simulink model "Control_Model_2020a"  (R2020a)
settings: Solver=ode3  StartTime=0.0  StopTime=20  FixedStep=0.001  RelTol=1e-3
InitFcn:
  | init_parameters
undefined symbols (not defined in the file): Bf, Bm, Br, DiscIntNeverNeededParam, f, g, hg, i_sw, I_tire, Iz, k1, k2, k3, K_LQR, kd_beta, kd_omega, ki_beta, ki_omega, kp_beta, kp_omega, L, Lf, Lm, Lr, m, magnitude, mb, mw, Mz_K, Pn_motor, r, sigbuilder_block, Tn_motor, v_obj, vx0, w0
libraries: simulink x2, Solver_SF x1, simulink_extras x1
(part 1 of 2)
settings Model: Creator=Qian  LastModifiedBy=Administrator
settings OptimizationCC: LifeSpan=inf
settings DebuggingCC: ArithmeticOperatorsInVariantConditions=warning
settings SFSimCC: CustomCodeUndefinedFunction=UseInterfaceOnly
settings RTWCC: GenCodeOnly=on
settings CodeAppCC: StateflowObjectComments=on

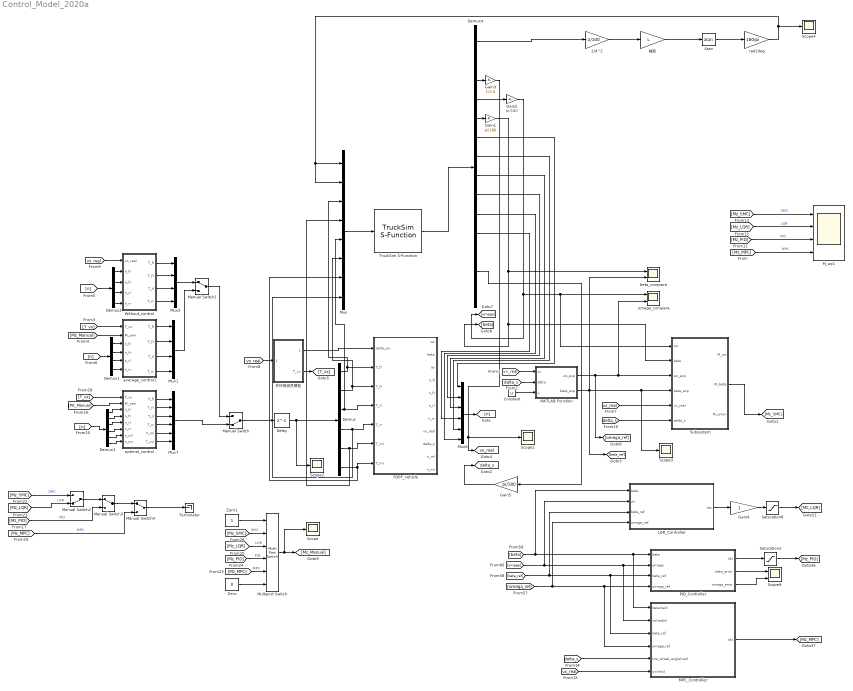
== system Control_Model_2020a ==
  2/d^2 : Gain  Gain=-2/100
  7DOF_vehicle : Subsystem
  Atan : Trigonometry  Operator=atan
  Constant : Constant  Value=u
  Delay : Delay  DelayLength=1
  Demux : Demux  Outputs=6
  Demux1 : Demux
  Demux2 : Demux
  Demux3 : Demux  Outputs=6
  Demux4 : Demux  Outputs=14
  Gain1 : Gain  Gain=pi/180
  Gain2 : Gain  Gain=pi/180
  Gain3 : Gain  Gain=1/3.6
  Gain4 : Gain
  Gain5 : Gain  Gain=pi/180
  LQR_Controller : Subsystem
  MATLAB Function : MATLAB Function  TreatAsAtomicUnit=on
  MPC_Controller : Subsystem
  M_wz1 : Scope  NumInputPorts=4
  Manual Switch : ManualSwitch  CurrentSetting=0
  Manual Switch1 : ManualSwitch
  Manual Switch2 : ManualSwitch  CurrentSetting=0
  Manual Switch3 : ManualSwitch
  Manual Switch4 : ManualSwitch
  Multiport Switch : MultiPortSwitch  Inputs=5
  Mux : Mux  Inputs=8
  Mux1 : Mux
  Mux3 : Mux
  Mux6 : Mux  Inputs=6
  Mux7 : Mux  Inputs=6
  PID_Controller : Subsystem
  Saturation2 : Saturate  UpperLimit=2000  LowerLimit=-2000
  Saturation8 : Saturate  UpperLimit=2000  LowerLimit=-2000
  Scope{,1..4} (5 alike) : Scope
  Scope9 : Scope  NumInputPorts=2
  Subsystem : Subsystem
  Terminator : Terminator
  TruckSim S-Function : Solver_SF/TruckSim S-Function  Priority=1  SIMFILE=simfile.sim
      settings: SourceProductName=TruckSim S-Function
  Without_control : Subsystem
  Zero : Constant  Value=0  OutDataTypeStr=Inherit: Inherit via back propagation
  Zero1 : Constant  OutDataTypeStr=Inherit: Inherit via back propagation
  average_control1 : Subsystem
  beta_compare : Scope  NumInputPorts=2
  omega_compare : Scope  NumInputPorts=2
  optimal_control : Subsystem
  rad2deg : Gain  Gain=180/pi
  开环驾驶员模型 : Subsystem
  轴距 : Gain  Gain=L
  tag scope: delta_s=global, vx_real=global
  wires:
  Demux2/1 -> Without_control/2(n_fl)
  Demux3/2 -> optimal_control/4(n_fr)
  [delta_s] -> MPC_Controller/5(tire_wheel_angle(rad))
  MPC_Controller/1(Mz) -> [Mz_MPC]
  Demux1/4 -> average_control1/6(n_rr)
  [n] -> Demux1/1
  [Mz_SMC] -> M_wz1/1  "SMC"
  PID_Controller/3(omega_error) -> Scope9/2
  Manual Switch/1 -> Delay/1
  MATLAB Function/2(beta_exp) -> [beta_ref], beta_compare/2, Scope3/1, Subsystem/4(beta_exp)
  average_control1/4(T_rr) -> Mux1/4
  Demux3/1 -> optimal_control/3(n_fl)
  Demux1/3 -> average_control1/5(n_rl)
  [Mz_Manual] -> average_control1/2(M_yaw)
  [n] -> Demux2/1
  average_control1/3(T_rl) -> Mux1/3
  Demux3/4 -> optimal_control/6(n_rr)
  Demux1/2 -> average_control1/4(n_fr)
  MATLAB Function/1(wz_exp) -> omega_compare/2, Subsystem/3(wz_exp), [omega_ref]
  开环驾驶员模型/1(delta_sw) -> 7DOF_vehicle/1(delta_sw)
  Demux/4 -> Mux/8, 7DOF_vehicle/5(T_rr)
  Demux/3 -> 7DOF_vehicle/4(T_rl), Mux/5
  Demux/1 -> Mux/3, 7DOF_vehicle/2(T_fl)
  Without_control/3(T_rl) -> Mux3/3
  Demux2/3 -> Without_control/4(n_rl)
  [n] -> Demux3/1
  Constant/1 -> MATLAB Function/3(u)
  optimal_control/2(T_fr) -> Mux7/2
  [vx_real] -> Without_control/1(vx_real)
  optimal_control/1(T_fl) -> Mux7/1
  Without_control/2(T_fr) -> Mux3/2
  Demux2/4 -> Without_control/5(n_rr)
  Demux2/2 -> Without_control/3(n_fr)
  Without_control/4(T_rr) -> Mux3/4
  Without_control/1(T_fl) -> Mux3/1
  Manual Switch4/1 -> Terminator/1
  average_control1/2(T_fr) -> Mux1/2
  [beta] -> LQR_Controller/1(beta), MPC_Controller/1(beta(rad)), PID_Controller/1(beta)
  Manual Switch3/1 -> Manual Switch4/1
  optimal_control/3(T_rl) -> Mux7/3
  [T_vx] -> optimal_control/1(T_vx)
  [Mz_Manual] -> optimal_control/2(M_yaw)
  [Mz_PID] -> Manual Switch3/2  "PID"
  [vx_real] -> MPC_Controller/6(vx(m/s))
  [vx_real] -> MATLAB Function/1(vx)
  [Mz_MPC] -> Manual Switch4/2  "MPC"
  [omega] -> LQR_Controller/2(wr), PID_Controller/2(omega), MPC_Controller/2(wr(rad/s))
  [vx_real] -> 开环驾驶员模型/1(vx_real)
  Saturation2/1 -> [Mz_PID]
  [Mz_SMC] -> Manual Switch2/1  "SMC"
  optimal_control/4(T_rr) -> Mux7/4
  Mux6/1 -> [n]
  Demux1/1 -> average_control1/3(n_fl)
  [T_vx] -> average_control1/1(T_vx)
  [omega_ref] -> LQR_Controller/4(omega_ref), PID_Controller/4(omega_ref), MPC_Controller/4(omega_ref)
  Mux7/1 -> Manual Switch/2
  LQR_Controller/1(Mz) -> Gain4/1
  [Mz_LQR] -> M_wz1/2  "LQR"
  PID_Controller/2(beta_error) -> Scope9/1
  [Mz_PID] -> M_wz1/3  "PID"
  Demux/2 -> Mux/6, 7DOF_vehicle/3(T_fr)
  Mux3/1 -> Manual Switch1/1
  average_control1/1(T_fl) -> Mux1/1
  [Mz_MPC] -> M_wz1/4  "MPC"
  Manual Switch2/1 -> Manual Switch3/1
  [beta_ref] -> LQR_Controller/3(beta_ref), PID_Controller/3(beta_ref), MPC_Controller/3(beta_ref)
  Mux1/1 -> Manual Switch1/2
  PID_Controller/1(Mz) -> Saturation2/1
  开环驾驶员模型/2(T_vx) -> [T_vx]
  [delta_s] -> MATLAB Function/2(delta)
  [Mz_LQR] -> Manual Switch2/2  "LQR"
  Demux3/3 -> optimal_control/5(n_rl)
  Manual Switch1/1 -> Manual Switch/1
  [Mz_SMC] -> Multiport Switch/2  "SMC"
  [Mz_MPC] -> Multiport Switch/5  "MPC"
  [Mz_PID] -> Multiport Switch/4  "PID"
  [Mz_LQR] -> Multiport Switch/3  "LQR"
  Zero/1 -> Multiport Switch/6
  Multiport Switch/1 -> Scope/1, [Mz_Manual]
  Zero1/1 -> Multiport Switch/1
  Saturation8/1 -> [Mz_LQR]
  Gain4/1 -> Saturation8/1
  Delay/1 -> Scope2/1, Demux/1
  optimal_control/5(T_ml) -> Mux7/5
  optimal_control/6(T_mr) -> Mux7/6
  Demux/5 -> Mux/4, 7DOF_vehicle/6(T_ml)
  Demux/6 -> Mux/7, 7DOF_vehicle/7(T_mr)
  Demux3/5 -> optimal_control/7(n_ml)
  Demux3/6 -> optimal_control/8(n_mr)
  TruckSim S-Function/1 -> Demux4/1
  Mux/1 -> TruckSim S-Function/1
  Demux4/4 -> Gain2/1
  Demux4/5 -> Gain1/1
  Demux4/6 -> Mux6/1
  Demux4/7 -> Mux6/5
  Demux4/8 -> Mux6/3
  Demux4/9 -> Mux6/2
  Demux4/10 -> Mux6/6
  Demux4/11 -> Mux6/4
  Demux4/3 -> Gain3/1
  2/d^2/1 -> 轴距/1
  轴距/1 -> Atan/1
  Atan/1 -> rad2deg/1
  Demux4/1 -> 2/d^2/1
  rad2deg/1 -> Scope4/1, Mux/1, Mux/2
  [delta_s] -> Subsystem/6(delta_s)
  [vx_real] -> Subsystem/5(vx_real)
  Gain3/1 -> Scope1/1, [vx_real]
  Gain1/1 -> beta_compare/1, [beta], Subsystem/2(beta)
  Gain2/1 -> [omega], Subsystem/1(wz), omega_compare/1
  Gain5/1 -> [delta_s]
  Demux4/13 -> Gain5/1
  Subsystem/2(M_beta) -> [Mz_SMC]

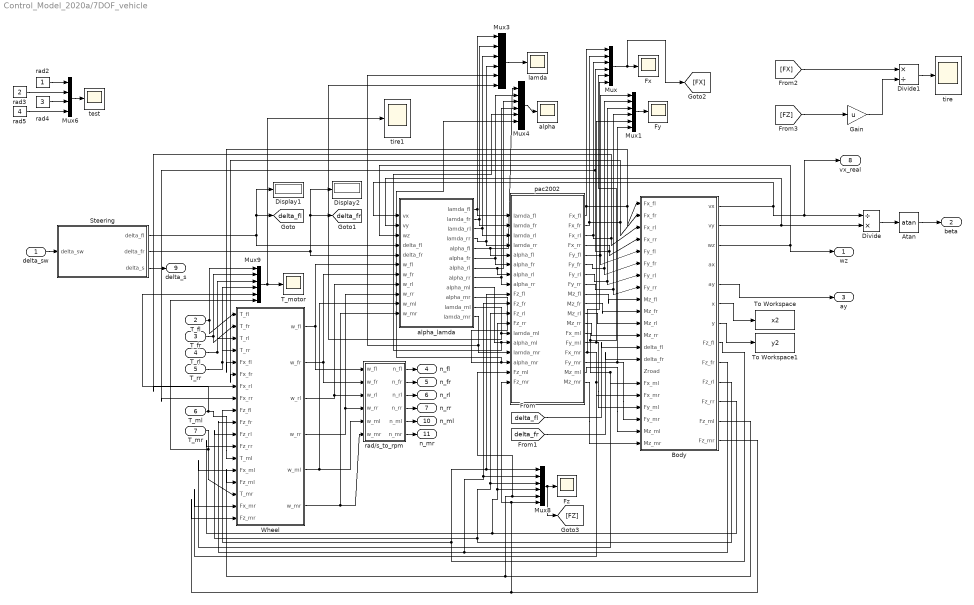
== system Control_Model_2020a/7DOF_vehicle ==
  delta_sw : Inport
  T_fl : Inport  Port=2
  T_fr : Inport  Port=3
  T_rl : Inport  Port=4
  T_rr : Inport  Port=5
  T_ml : Inport  Port=6
  T_mr : Inport  Port=7
  Atan : Trigonometry  Operator=atan
  Body : Subsystem
  Display1 : Display
  Display2 : Display
  Divide : Product  Inputs=/*
  Divide1 : Product  Inputs=*/
  Fx : Scope
  Fy : Scope
  Fz : Scope
  Gain : Gain  Gain=u
  Mux{,1,3..4,8..9} (6 alike) : Mux  Inputs=6
  Mux6 : Mux
  Steering : Subsystem
  T_motor : Scope
  To Workspace : ToWorkspace  VariableName=x2  SampleTime=-1
  To Workspace1 : ToWorkspace  VariableName=y2  SampleTime=-1
  Wheel : Subsystem
  alpha : Scope
  alpha_lamda : Subsystem
  lamda : Scope
  pac2002 : Subsystem
  rad/s_to_rpm : Subsystem
  rad2 : Constant
  rad3 : Constant  Value=2
  rad4 : Constant  Value=3
  rad5 : Constant  Value=4
  test : Scope
  tire : Scope
  tire1 : Scope
  wz : Outport
  beta : Outport  Port=2
  ay : Outport  Port=3
  n_fl : Outport  Port=4
  n_fr : Outport  Port=5
  n_rl : Outport  Port=6
  n_rr : Outport  Port=7
  vx_real : Outport  Port=8
  delta_s : Outport  Port=9
  n_ml : Outport  Port=10
  n_mr : Outport  Port=11
  tag scope: delta_fl=global, delta_fr=global
  wires:
  pac2002/12(Mz_rr) -> Body/12(Mz_rr)
  pac2002/11(Mz_rl) -> Body/11(Mz_rl)
  pac2002/10(Mz_fr) -> Body/10(Mz_fr)
  pac2002/9(Mz_fl) -> Body/9(Mz_fl)
  Atan/1 -> beta/1
  Divide/1 -> Atan/1
  T_rr/1 -> Mux9/4, Wheel/4(T_rr)
  rad/s_to_rpm/4(n_rr) -> n_rr/1
  rad/s_to_rpm/2(n_fr) -> n_fr/1
  T_rl/1 -> Mux9/3, Wheel/3(T_rl)
  Body/5(ay) -> ay/1
  Body/1(vx) -> vx_real/1, Divide/1, alpha_lamda/1(vx)
  Mux6/1 -> test/1
  Wheel/4(w_rr) -> alpha_lamda/9(w_rr), rad/s_to_rpm/4(w_rr)
  rad3/1 -> Mux6/2
  delta_sw/1 -> Steering/1(delta_sw)
  Body/2(vy) -> alpha_lamda/2(vy), Divide/2
  rad4/1 -> Mux6/3
  rad5/1 -> Mux6/4
  Mux3/1 -> lamda/1
  Mux/1 -> [FX], Fx/1
  T_fl/1 -> Mux9/1, Wheel/1(T_fl)
  Body/11(Fz_rr) -> pac2002/12(Fz_rr), Mux8/4, Wheel/12(Fz_rr)
  Mux4/1 -> alpha/1
  rad/s_to_rpm/3(n_rl) -> n_rl/1
  T_fr/1 -> Mux9/2, Wheel/2(T_fr)
  pac2002/3(Fx_rl) -> Mux/3, Body/3(Fx_rl), Wheel/7(Fx_rl)
  alpha_lamda/6(alpha_fr) -> pac2002/6(alpha_fr), Mux4/2
  Body/9(Fz_fr) -> pac2002/10(Fz_fr), Mux8/2, Wheel/10(Fz_fr)
  [delta_fr] -> Body/14(delta_fr)
  alpha_lamda/5(alpha_fl) -> pac2002/5(alpha_fl), Mux4/1
  alpha_lamda/8(alpha_rr) -> pac2002/8(alpha_rr), Mux4/4
  Wheel/1(w_fl) -> rad/s_to_rpm/1(w_fl), alpha_lamda/6(w_fl)
  Wheel/3(w_rl) -> rad/s_to_rpm/3(w_rl), alpha_lamda/8(w_rl)
  Body/10(Fz_rl) -> pac2002/11(Fz_rl), Mux8/3, Wheel/11(Fz_rl)
  Mux1/1 -> Fy/1
  rad/s_to_rpm/1(n_fl) -> n_fl/1
  alpha_lamda/7(alpha_rl) -> pac2002/7(alpha_rl), Mux4/3
  Mux8/1 -> [FZ], Fz/1
  Wheel/2(w_fr) -> rad/s_to_rpm/2(w_fr), alpha_lamda/7(w_fr)
  pac2002/8(Fy_rr) -> Body/8(Fy_rr), Mux1/4
  alpha_lamda/2(lamda_fr) -> pac2002/2(lamda_fr), Mux3/2
  pac2002/5(Fy_fl) -> Body/5(Fy_fl), Mux1/1
  pac2002/2(Fx_fr) -> Mux/2, Body/2(Fx_fr), Wheel/6(Fx_fr)
  Body/8(Fz_fl) -> pac2002/9(Fz_fl), Mux8/1, Wheel/9(Fz_fl)
  alpha_lamda/3(lamda_rl) -> pac2002/3(lamda_rl), Mux3/3
  pac2002/6(Fy_fr) -> Body/6(Fy_fr), Mux1/2
  pac2002/7(Fy_rl) -> Body/7(Fy_rl), Mux1/3
  Steering/2(delta_fr) -> alpha_lamda/5(delta_fr), Display2/1, [delta_fr]
  Steering/1(delta_fl) -> alpha_lamda/4(delta_fl), Display1/1, [delta_fl]
  alpha_lamda/4(lamda_rr) -> pac2002/4(lamda_rr), Mux3/4
  alpha_lamda/1(lamda_fl) -> Mux3/1, pac2002/1(lamda_fl)
  pac2002/1(Fx_fl) -> Mux/1, Body/1(Fx_fl), Wheel/5(Fx_fl)
  rad2/1 -> Mux6/1
  [delta_fl] -> Body/13(delta_fl)
  Body/3(wz) -> wz/1, alpha_lamda/3(wz)
  pac2002/4(Fx_rr) -> Mux/4, Wheel/8(Fx_rr), Body/4(Fx_rr)
  Body/6(x) -> To Workspace/1
  Body/7(y) -> To Workspace1/1
  [FZ] -> Gain/1
  [FX] -> Divide1/1
  Gain/1 -> Divide1/2
  Divide1/1 -> tire/1
  Mux9/1 -> tire1/1, T_motor/1
  Steering/3(delta_s) -> delta_s/1
  rad/s_to_rpm/5(n_ml) -> n_ml/1
  rad/s_to_rpm/6(n_mr) -> n_mr/1
  Wheel/5(w_ml) -> alpha_lamda/10(w_ml), rad/s_to_rpm/5(w_ml)
  Wheel/6(w_mr) -> alpha_lamda/11(w_mr), rad/s_to_rpm/6(w_mr)
  alpha_lamda/11(lamda_ml) -> Mux3/6, pac2002/13(lamda_ml)
  alpha_lamda/9(alpha_ml) -> Mux4/5, pac2002/14(alpha_ml)
  alpha_lamda/10(alpha_mr) -> Mux4/6, pac2002/16(alpha_mr)
  alpha_lamda/12(lamda_mr) -> Mux3/5, pac2002/15(lamda_mr)
  Body/12(Fz_ml) -> Wheel/15(Fz_ml), pac2002/17(Fz_ml), Mux8/5
  Body/13(Fz_mr) -> Wheel/18(Fz_mr), Mux8/6, pac2002/18(Fz_mr)
  pac2002/13(Fx_ml) -> Mux/5, Wheel/14(Fx_ml), Body/16(Fx_ml)
  pac2002/15(Fx_mr) -> Mux/6, Wheel/17(Fx_mr), Body/17(Fx_mr)
  pac2002/16(Fy_mr) -> Body/19(Fy_mr), Mux1/6
  pac2002/14(Fy_ml) -> Body/18(Fy_ml), Mux1/5
  pac2002/17(Mz_ml) -> Body/20(Mz_ml)
  pac2002/18(Mz_mr) -> Body/21(Mz_mr)
  T_ml/1 -> Wheel/13(T_ml), Mux9/5
  T_mr/1 -> Mux9/6, Wheel/16(T_mr)

== system Control_Model_2020a/LQR_Controller ==
  beta : Inport
  wr : Inport  Port=2
  beta_ref : Inport  Port=3
  omega_ref : Inport  Port=4
  Add2 : Sum  Inputs=+-
  Add7 : Sum  Inputs=+-
  Add8 : Sum
  Gain1 : Gain  Gain=-K_LQR(2)
  Gain2 : Gain  Gain=-K_LQR(1)
  Mz : Outport
  wires:
  Add2/1 -> Gain2/1
  Gain1/1 -> Add8/1
  beta_ref/1 -> Add2/2
  wr/1 -> Add7/1
  omega_ref/1 -> Add7/2
  Gain2/1 -> Add8/2
  beta/1 -> Add2/1
  Add7/1 -> Gain1/1
  Add8/1 -> Mz/1

== system Control_Model_2020a/MPC_Controller ==
  beta(rad) : Inport
  wr(rad/s) : Inport  Port=2
  beta_ref : Inport  Port=3
  omega_ref : Inport  Port=4
  tire_wheel_angle(rad) : Inport  Port=5
  vx(m/s) : Inport  Port=6
  Constant16 : Constant  Value=0.01
  Delay2 : Delay  DelayLength=1
  MATLAB Function : MATLAB Function  TreatAsAtomicUnit=on
  Mux4 : Mux  Inputs=8
  Mz : Outport
  wires:
  beta(rad)/1 -> Mux4/1  "质心侧偏角"
  tire_wheel_angle(rad)/1 -> Mux4/3  "车轮转角"
  vx(m/s)/1 -> Mux4/4  "车速"
  Mux4/1 -> MATLAB Function/1(x)
  wr(rad/s)/1 -> Mux4/2  "横摆角速度"
  beta_ref/1 -> Mux4/5
  omega_ref/1 -> Mux4/6
  Delay2/1 -> Mux4/8
  Constant16/1 -> Mux4/7
  MATLAB Function/1(delta_u) -> Delay2/1, Mz/1

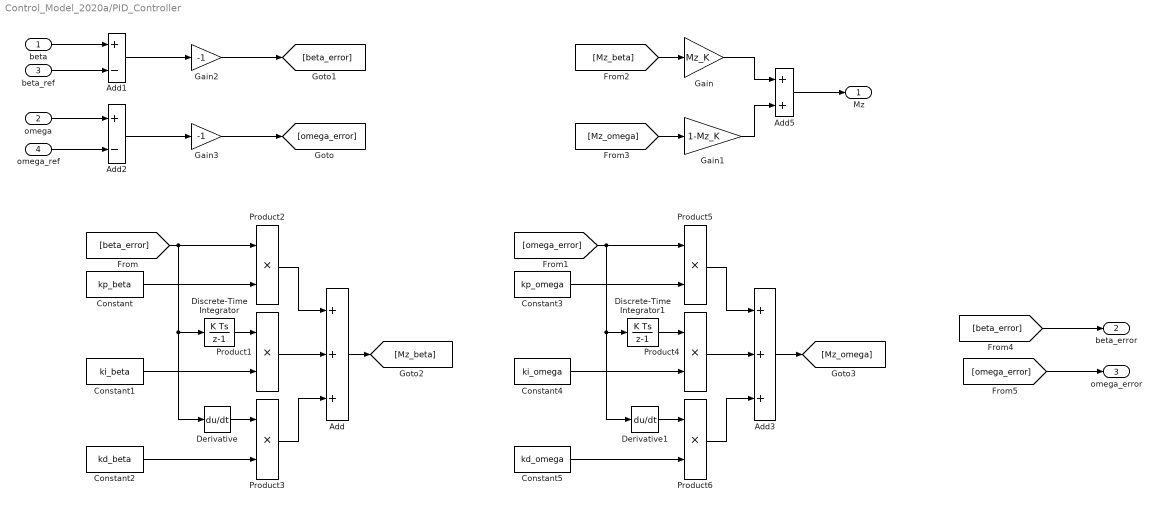
== system Control_Model_2020a/PID_Controller ==
  beta : Inport
  omega : Inport  Port=2
  beta_ref : Inport  Port=3
  omega_ref : Inport  Port=4
  Add : Sum  Inputs=+++
  Add1 : Sum  Inputs=+-
  Add2 : Sum  Inputs=+-
  Add3 : Sum  Inputs=+++
  Add5 : Sum  Inputs=2
  Constant : Constant  Value=kp_beta
  Constant1 : Constant  Value=ki_beta
  Constant2 : Constant  Value=kd_beta
  Constant3 : Constant  Value=kp_omega
  Constant4 : Constant  Value=ki_omega
  Constant5 : Constant  Value=kd_omega
  Derivative : Derivative
  Derivative1 : Derivative
  Discrete-Time Integrator : DiscreteIntegrator  SampleTime=-1  ICPrevOutput=DiscIntNeverNeededParam  ICPrevScaledInput=DiscIntNeverNeededParam
  Discrete-Time Integrator1 : DiscreteIntegrator  SampleTime=-1  ICPrevOutput=DiscIntNeverNeededParam  ICPrevScaledInput=DiscIntNeverNeededParam
  Gain : Gain  Gain=Mz_K
  Gain1 : Gain  Gain=1-Mz_K
  Gain2 : Gain  Gain=-1
  Gain3 : Gain  Gain=-1
  Product{1..6} (6 alike) : Product
  Mz : Outport
  beta_error : Outport  Port=2
  omega_error : Outport  Port=3
  wires:
  Add2/1 -> Gain3/1
  beta/1 -> Add1/1
  omega_ref/1 -> Add2/2
  beta_ref/1 -> Add1/2
  omega/1 -> Add2/1
  Add1/1 -> Gain2/1
  [beta_error] -> Product2/1, Discrete-Time Integrator/1, Derivative/1
  Constant/1 -> Product2/2
  Product2/1 -> Add/1
  Constant1/1 -> Product1/2
  Discrete-Time Integrator/1 -> Product1/1
  Constant2/1 -> Product3/2
  Derivative/1 -> Product3/1
  Product1/1 -> Add/2
  Product3/1 -> Add/3
  Product5/1 -> Add3/1
  Discrete-Time Integrator1/1 -> Product4/1
  [omega_error] -> Product5/1, Discrete-Time Integrator1/1, Derivative1/1
  Constant5/1 -> Product6/2
  Product6/1 -> Add3/3
  Constant4/1 -> Product4/2
  Constant3/1 -> Product5/2
  Derivative1/1 -> Product6/1
  Product4/1 -> Add3/2
  Add/1 -> [Mz_beta]
  Add3/1 -> [Mz_omega]
  [Mz_beta] -> Gain/1
  Add5/1 -> Mz/1
  Gain/1 -> Add5/1
  [Mz_omega] -> Gain1/1
  Gain1/1 -> Add5/2
  Gain2/1 -> [beta_error]
  Gain3/1 -> [omega_error]
  [beta_error] -> beta_error/1
  [omega_error] -> omega_error/1

== system Control_Model_2020a/Subsystem ==
  note: 这里有个比例环节，是为了缩小所求的M_wz,
      | 同时也降低扭矩输出变化率，可根据实际调试情况调整
  wz : Inport
  beta : Inport  Port=2
  wz_exp : Inport  Port=3
  beta_exp : Inport  Port=4
  vx_real : Inport  Port=5
  delta_s : Inport  Port=6
  Constant : Constant  Value=u
  Constant1 : Constant
  Controller_beta : Subsystem
  Controller_wz : Subsystem
  Product : Product
  Product1 : Product
  Scope : Scope
  Sum1 : Sum  Inputs=|++
  Sum2 : Sum  Inputs=+-|
  Union_Control : Subsystem
  比例环节1 : Gain  Gain=1/6
  比例环节2 : Gain  Gain=1/6.3
  M_wz : Outport
  M_beta : Outport  Port=2
  M_union : Outport  Port=3
  wires:
  beta/1 -> Controller_wz/3(beta), Controller_beta/3(beta), Union_Control/1(beta)
  wz/1 -> Controller_wz/1(wz), Controller_beta/1(wz)
  wz_exp/1 -> Controller_wz/2(wz_exp)
  beta_exp/1 -> Controller_beta/2(beta_exp)
  Controller_wz/1(M_wz) -> 比例环节1/1
  Controller_beta/1(M_beta) -> 比例环节2/1
  vx_real/1 -> Controller_beta/5(vx), Controller_wz/4(vx)
  delta_s/1 -> Controller_beta/4(delta_s), Controller_wz/5(delta_s)
  比例环节1/1 -> Product/2, M_wz/1
  比例环节2/1 -> Product1/2, M_beta/1
  Union_Control/1(p) -> Product1/1, Sum2/2, Scope/1
  Constant1/1 -> Sum2/1
  Sum2/1 -> Product/1
  Product/1 -> Sum1/1
  Sum1/1 -> M_union/1
  Product1/1 -> Sum1/2
  Constant/1 -> Union_Control/2(u)

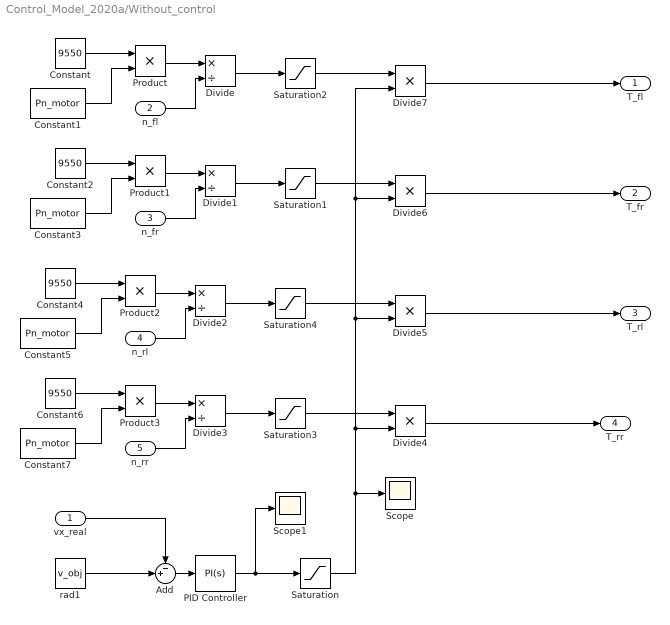
== system Control_Model_2020a/Without_control ==
  vx_real : Inport
  n_fl : Inport  Port=2
  n_fr : Inport  Port=3
  n_rl : Inport  Port=4
  n_rr : Inport  Port=5
  Add : Sum  Inputs=-+|
  Constant{,2,4,6} (4 alike) : Constant  Value=9550
  Constant{1,3,5,7} (4 alike) : Constant  Value=Pn_motor
  Divide{,1..3} (4 alike) : Product  Inputs=*/
  Divide{4..7} (4 alike) : Product  Inputs=**
  PID Controller : simulink/Continuous/PID Controller  Controller=PI  Form=Parallel  TimeDomain=Continuous-time  UseExternalTs=off  SampleTime=1  IntegratorMethod=Forward Euler  FilterMethod=Forward Euler  ControllerParametersSource=internal  P=1  I=0  D=0  UseFilter=on  N=100  TunerSelectOption=Transfer Function Based (PID Tuner App)  InitialConditionSource=internal  InitialConditionForIntegrator=0  InitialConditionForFilter=0  DifferentiatorICPrevScaledInput=0  ExternalReset=none  TrackingMode=off  Kt=1  LimitOutput=off  UpperSaturationLimit=inf  LowerSaturationLimit=-inf  LinearizeAsGain=on  AntiWindupMode=none  Kb=1  POutMin=[]  POutMax=[]  IOutMin=[]  IOutMax=[]  DOutMin=[]  DOutMax=[]  NOutMin=[]  NOutMax=[]  SumOutMin=[]  SumOutMax=[]  SaturationOutMin=[]  SaturationOutMax=[]  PParamMin=[]  PParamMax=[]  IParamMin=[]  IParamMax=[]  DParamMin=[]  DParamMax=[]  NParamMin=[]  NParamMax=[]  KbParamMin=[]  KbParamMax=[]  KtParamMin=[]  KtParamMax=[]  KbOutMin=[]  KbOutMax=[]  KtOutMin=[]  KtOutMax=[]  IntegratorOutMin=[]  IntegratorOutMax=[]  FilterOutMin=[]  FilterOutMax=[]  SumI1OutMin=[]  SumI1OutMax=[]  SumI2OutMin=[]  SumI2OutMax=[]  SumI3OutMin=[]  SumI3OutMax=[]  SumI4OutMin=[]  SumI4OutMax=[]  SumDOutMin=[]  SumDOutMax=[]  DifferentiatorOutMin=[]  DifferentiatorOutMax=[]  FilterDiffOutCoefMin=[]  FilterDiffOutCoefMax=[]  ReciprocalOutMin=[]  ReciprocalOutMax=[]  SumDenOutMin=[]  SumDenOutMax=[]  SumNumOutMin=[]  SumNumOutMax=[]  DivideOutMin=[]  DivideOutMax=[]  UdiffTsProdOutMin=[]  UdiffTsProdOutMax=[]  NTsProdOutMin=[]  NTsProdOutMax=[]  UintegralTsProdOutMin=[]  UintegralTsProdOutMax=[]  UngainTsProdOutMin=[]  UngainTsProdOutMax=[]  IntegratorContinuousStateAttributes=''  IntegratorStateMustResolveToSignalObject=off  IntegratorRTWStateStorageClass=Auto  FilterContinuousStateAttributes=''  FilterStateMustResolveToSignalObject=off  FilterRTWStateStorageClass=Auto  ParallelPVariant=InternalParameters  IdealPVariant=Disabled  IVariant=InternalParameters  DVariant=Disabled  IntegratorVariant=Continuous  SatVariant=Disabled  AWVariant=Passthrough  PCopyVariant=Disabled  TRVariant=Disabled  FdbkBlocksVariant=Forward  IdealPFdbkVariant=Disabled  SatFdbkVariant=Disabled  DerivativeFilterVariant=Disabled  NVariant=Disabled  NCopyVariant=Disabled_SignalSpec  FilterICVariant=Disabled  IntegratorICVariant=InternalICs  ExternalResetVariant=Disabled  TRSumVariant=Passthrough  SumFdbkVariant=Disabled  SumVariant=Sum_PI  TsampFilterVariant=InternalTs  TsampNgainVariant=Passthrough  TsampIntegralVariant=Passthrough
  Product{,1..3} (4 alike) : Product
  Saturation : Saturate  UpperLimit=1  LowerLimit=-1
  Saturation{1..4} (4 alike) : Saturate  UpperLimit=Tn_motor  LowerLimit=-Tn_motor
  Scope : Scope
  Scope1 : Scope
  rad1 : Constant  Value=v_obj
  T_fl : Outport
  T_fr : Outport  Port=2
  T_rl : Outport  Port=3
  T_rr : Outport  Port=4
  wires:
  Saturation/1 -> Divide7/2, Divide6/2, Divide5/2, Divide4/2, Scope/1
  Add/1 -> PID Controller/1
  rad1/1 -> Add/2
  PID Controller/1 -> Saturation/1, Scope1/1
  Divide4/1 -> T_rr/1
  Divide5/1 -> T_rl/1
  Divide6/1 -> T_fr/1
  Divide7/1 -> T_fl/1
  vx_real/1 -> Add/1
  n_fl/1 -> Divide/2
  Divide/1 -> Saturation2/1
  Constant/1 -> Product/1
  Constant1/1 -> Product/2
  Product/1 -> Divide/1
  n_fr/1 -> Divide1/2
  Divide1/1 -> Saturation1/1
  Constant2/1 -> Product1/1
  Constant3/1 -> Product1/2
  Product1/1 -> Divide1/1
  n_rl/1 -> Divide2/2
  Divide2/1 -> Saturation4/1
  Constant4/1 -> Product2/1
  Constant5/1 -> Product2/2
  Product2/1 -> Divide2/1
  n_rr/1 -> Divide3/2
  Divide3/1 -> Saturation3/1
  Constant6/1 -> Product3/1
  Constant7/1 -> Product3/2
  Product3/1 -> Divide3/1
  Saturation3/1 -> Divide4/1
  Saturation4/1 -> Divide5/1
  Saturation1/1 -> Divide6/1
  Saturation2/1 -> Divide7/1

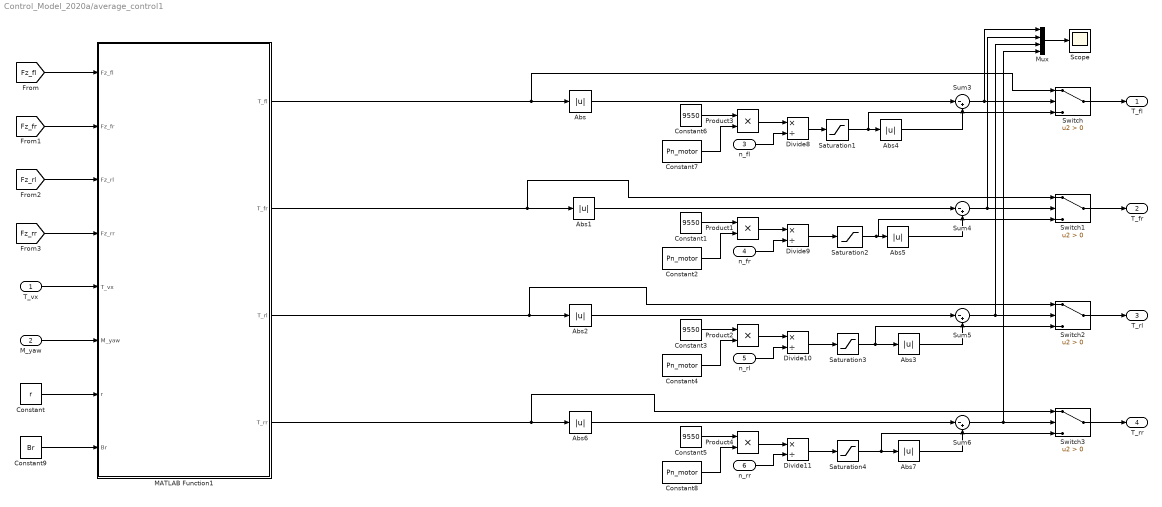
== system Control_Model_2020a/average_control1 ==
  T_vx : Inport
  M_yaw : Inport  Port=2
  n_fl : Inport  Port=3
  n_fr : Inport  Port=4
  n_rl : Inport  Port=5
  n_rr : Inport  Port=6
  Abs{,1..7} (8 alike) : Abs
  Constant : Constant  Value=r
  Constant{1,3,5..6} (4 alike) : Constant  Value=9550
  Constant{2,4,7..8} (4 alike) : Constant  Value=Pn_motor
  Constant9 : Constant  Value=Br
  Divide{8..11} (4 alike) : Product  Inputs=*/
  MATLAB Function1 : MATLAB Function  TreatAsAtomicUnit=on
  Mux : Mux
  Product{1..4} (4 alike) : Product
  Saturation{1..4} (4 alike) : Saturate  UpperLimit=Tn_motor  LowerLimit=-Tn_motor
  Scope : Scope
  Sum{3..6} (4 alike) : Sum  Inputs=|-+
  Switch{,1..3} (4 alike) : Switch  Criteria=u2 > Threshold
  T_fl : Outport
  T_fr : Outport  Port=2
  T_rl : Outport  Port=3
  T_rr : Outport  Port=4
  wires:
  MATLAB Function1/4(T_rr) -> Abs6/1, Switch3/1
  MATLAB Function1/3(T_rl) -> Abs2/1, Switch2/1
  MATLAB Function1/2(T_fr) -> Abs1/1, Switch1/1
  MATLAB Function1/1(T_fl) -> Abs/1, Switch/1
  Mux/1 -> Scope/1
  Constant9/1 -> MATLAB Function1/8(Br)
  Constant/1 -> MATLAB Function1/7(r)
  M_yaw/1 -> MATLAB Function1/6(M_yaw)
  T_vx/1 -> MATLAB Function1/5(T_vx)
  [Fz_rr] -> MATLAB Function1/4(Fz_rr)
  [Fz_fr] -> MATLAB Function1/2(Fz_fr)
  [Fz_rl] -> MATLAB Function1/3(Fz_rl)
  [Fz_fl] -> MATLAB Function1/1(Fz_fl)
  Saturation4/1 -> Switch3/3, Abs7/1
  Saturation3/1 -> Abs3/1, Switch2/3
  Saturation1/1 -> Abs4/1, Switch/3
  Saturation2/1 -> Switch1/3, Abs5/1
  Constant5/1 -> Product4/1
  Constant8/1 -> Product4/2
  Product4/1 -> Divide11/1
  Divide11/1 -> Saturation4/1
  Abs6/1 -> Sum6/1
  Abs7/1 -> Sum6/2
  Sum6/1 -> Switch3/2, Mux/4
  Switch3/1 -> T_rr/1
  n_rr/1 -> Divide11/2
  n_rl/1 -> Divide10/2
  Switch2/1 -> T_rl/1
  Sum5/1 -> Switch2/2, Mux/3
  Abs3/1 -> Sum5/2
  Abs2/1 -> Sum5/1
  Divide10/1 -> Saturation3/1
  Product2/1 -> Divide10/1
  Constant4/1 -> Product2/2
  Constant3/1 -> Product2/1
  Constant1/1 -> Product1/1
  Constant2/1 -> Product1/2
  Product1/1 -> Divide9/1
  Divide9/1 -> Saturation2/1
  Abs1/1 -> Sum4/1
  Abs5/1 -> Sum4/2
  Sum4/1 -> Switch1/2, Mux/2
  Switch1/1 -> T_fr/1
  n_fr/1 -> Divide9/2
  n_fl/1 -> Divide8/2
  Switch/1 -> T_fl/1
  Sum3/1 -> Switch/2, Mux/1
  Abs4/1 -> Sum3/2
  Abs/1 -> Sum3/1
  Divide8/1 -> Saturation1/1
  Product3/1 -> Divide8/1
  Constant7/1 -> Product3/2
  Constant6/1 -> Product3/1

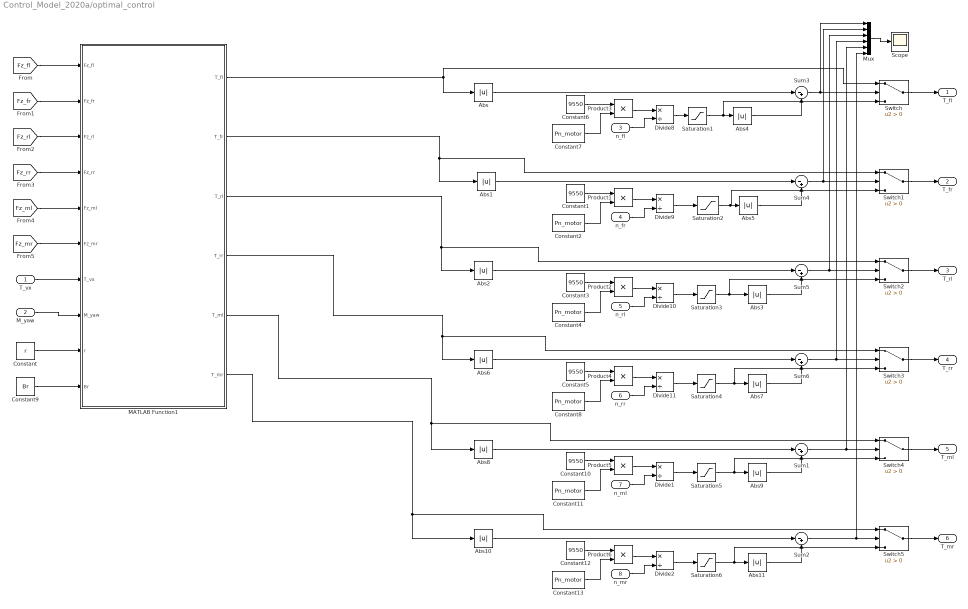
== system Control_Model_2020a/optimal_control ==
  T_vx : Inport
  M_yaw : Inport  Port=2
  n_fl : Inport  Port=3
  n_fr : Inport  Port=4
  n_rl : Inport  Port=5
  n_rr : Inport  Port=6
  n_ml : Inport  Port=7
  n_mr : Inport  Port=8
  Abs{,1..11} (12 alike) : Abs
  Constant : Constant  Value=r
  Constant{1,3,5..6,10,12} (6 alike) : Constant  Value=9550
  Constant{2,4,7..8,11,13} (6 alike) : Constant  Value=Pn_motor
  Constant9 : Constant  Value=Br
  Divide{1..2,8..11} (6 alike) : Product  Inputs=*/
  MATLAB Function1 : MATLAB Function  TreatAsAtomicUnit=on
  Mux : Mux  Inputs=6
  Product{1..6} (6 alike) : Product
  Saturation{1..6} (6 alike) : Saturate  UpperLimit=Tn_motor  LowerLimit=-Tn_motor
  Scope : Scope
  Sum{1..6} (6 alike) : Sum  Inputs=|-+
  Switch{,1..5} (6 alike) : Switch  Criteria=u2 > Threshold
  T_fl : Outport
  T_fr : Outport  Port=2
  T_rl : Outport  Port=3
  T_rr : Outport  Port=4
  T_ml : Outport  Port=5
  T_mr : Outport  Port=6
  wires:
  Constant6/1 -> Product3/1
  Constant7/1 -> Product3/2
  Product3/1 -> Divide8/1
  Divide8/1 -> Saturation1/1
  Abs/1 -> Sum3/1
  Abs4/1 -> Sum3/2
  Sum3/1 -> Mux/1, Switch/2
  Switch/1 -> T_fl/1
  n_fl/1 -> Divide8/2
  n_fr/1 -> Divide9/2
  Switch1/1 -> T_fr/1
  Sum4/1 -> Mux/2, Switch1/2
  Abs5/1 -> Sum4/2
  Abs1/1 -> Sum4/1
  Divide9/1 -> Saturation2/1
  Product1/1 -> Divide9/1
  Constant2/1 -> Product1/2
  Constant1/1 -> Product1/1
  Constant3/1 -> Product2/1
  Constant4/1 -> Product2/2
  Product2/1 -> Divide10/1
  Divide10/1 -> Saturation3/1
  Abs2/1 -> Sum5/1
  Abs3/1 -> Sum5/2
  Sum5/1 -> Mux/3, Switch2/2
  Switch2/1 -> T_rl/1
  n_rl/1 -> Divide10/2
  n_rr/1 -> Divide11/2
  Switch3/1 -> T_rr/1
  Sum6/1 -> Mux/4, Switch3/2
  Abs7/1 -> Sum6/2
  Abs6/1 -> Sum6/1
  Divide11/1 -> Saturation4/1
  Product4/1 -> Divide11/1
  Constant8/1 -> Product4/2
  Constant5/1 -> Product4/1
  Saturation2/1 -> Abs5/1, Switch1/3
  Saturation1/1 -> Switch/3, Abs4/1
  Saturation3/1 -> Switch2/3, Abs3/1
  Saturation4/1 -> Abs7/1, Switch3/3
  [Fz_fl] -> MATLAB Function1/1(Fz_fl)
  [Fz_rl] -> MATLAB Function1/3(Fz_rl)
  [Fz_fr] -> MATLAB Function1/2(Fz_fr)
  [Fz_rr] -> MATLAB Function1/4(Fz_rr)
  T_vx/1 -> MATLAB Function1/7(T_vx)
  M_yaw/1 -> MATLAB Function1/8(M_yaw)
  Constant/1 -> MATLAB Function1/9(r)
  Constant9/1 -> MATLAB Function1/10(Br)
  Mux/1 -> Scope/1
  MATLAB Function1/1(T_fl) -> Abs/1, Switch/1
  MATLAB Function1/2(T_fr) -> Abs1/1, Switch1/1
  MATLAB Function1/3(T_rl) -> Abs2/1, Switch2/1
  MATLAB Function1/4(T_rr) -> Abs6/1, Switch3/1
  Constant11/1 -> Product5/2
  Divide1/1 -> Saturation5/1
  Saturation5/1 -> Abs9/1, Switch4/3
  Sum1/1 -> Mux/5, Switch4/2
  Product5/1 -> Divide1/1
  Abs8/1 -> Sum1/1
  Constant10/1 -> Product5/1
  Abs9/1 -> Sum1/2
  Switch4/1 -> T_ml/1
  n_ml/1 -> Divide1/2
  Saturation6/1 -> Abs11/1, Switch5/3
  Divide2/1 -> Saturation6/1
  Constant13/1 -> Product6/2
  Switch5/1 -> T_mr/1
  n_mr/1 -> Divide2/2
  Product6/1 -> Divide2/1
  Sum2/1 -> Mux/6, Switch5/2
  Abs11/1 -> Sum2/2
  Constant12/1 -> Product6/1
  Abs10/1 -> Sum2/1
  MATLAB Function1/5(T_ml) -> Switch4/1, Abs8/1
  MATLAB Function1/6(T_mr) -> Switch5/1, Abs10/1
  [Fz_ml] -> MATLAB Function1/5(Fz_ml)
  [Fz_mr] -> MATLAB Function1/6(Fz_mr)

== system Control_Model_2020a/开环驾驶员模型 ==
  vx_real : Inport
  Add : Sum  Inputs=-+|
  DLC : Subsystem
  Gain : Gain  Gain=3.6
  Gain1 : Gain  Gain=3.6
  PID Controller : simulink/Continuous/PID Controller  Controller=PI  Form=Parallel  TimeDomain=Continuous-time  UseExternalTs=off  SampleTime=1  IntegratorMethod=Forward Euler  FilterMethod=Forward Euler  ControllerParametersSource=internal  P=2000  I=230  D=0  UseFilter=on  N=100  TunerSelectOption=Transfer Function Based (PID Tuner App)  InitialConditionSource=internal  InitialConditionForIntegrator=0  InitialConditionForFilter=0  DifferentiatorICPrevScaledInput=0  ExternalReset=none  TrackingMode=off  Kt=1  LimitOutput=off  UpperSaturationLimit=inf  LowerSaturationLimit=-inf  LinearizeAsGain=on  AntiWindupMode=none  Kb=1  POutMin=[]  POutMax=[]  IOutMin=[]  IOutMax=[]  DOutMin=[]  DOutMax=[]  NOutMin=[]  NOutMax=[]  SumOutMin=[]  SumOutMax=[]  SaturationOutMin=[]  SaturationOutMax=[]  PParamMin=[]  PParamMax=[]  IParamMin=[]  IParamMax=[]  DParamMin=[]  DParamMax=[]  NParamMin=[]  NParamMax=[]  KbParamMin=[]  KbParamMax=[]  KtParamMin=[]  KtParamMax=[]  KbOutMin=[]  KbOutMax=[]  KtOutMin=[]  KtOutMax=[]  IntegratorOutMin=[]  IntegratorOutMax=[]  FilterOutMin=[]  FilterOutMax=[]  SumI1OutMin=[]  SumI1OutMax=[]  SumI2OutMin=[]  SumI2OutMax=[]  SumI3OutMin=[]  SumI3OutMax=[]  SumI4OutMin=[]  SumI4OutMax=[]  SumDOutMin=[]  SumDOutMax=[]  DifferentiatorOutMin=[]  DifferentiatorOutMax=[]  FilterDiffOutCoefMin=[]  FilterDiffOutCoefMax=[]  ReciprocalOutMin=[]  ReciprocalOutMax=[]  SumDenOutMin=[]  SumDenOutMax=[]  SumNumOutMin=[]  SumNumOutMax=[]  DivideOutMin=[]  DivideOutMax=[]  UdiffTsProdOutMin=[]  UdiffTsProdOutMax=[]  NTsProdOutMin=[]  NTsProdOutMax=[]  UintegralTsProdOutMin=[]  UintegralTsProdOutMax=[]  UngainTsProdOutMin=[]  UngainTsProdOutMax=[]  IntegratorContinuousStateAttributes=''  IntegratorStateMustResolveToSignalObject=off  IntegratorRTWStateStorageClass=Auto  FilterContinuousStateAttributes=''  FilterStateMustResolveToSignalObject=off  FilterRTWStateStorageClass=Auto  ParallelPVariant=InternalParameters  IdealPVariant=Disabled  IVariant=InternalParameters  DVariant=Disabled  IntegratorVariant=Continuous  SatVariant=Disabled  AWVariant=Passthrough  PCopyVariant=Disabled  TRVariant=Disabled  FdbkBlocksVariant=Forward  IdealPFdbkVariant=Disabled  SatFdbkVariant=Disabled  DerivativeFilterVariant=Disabled  NVariant=Disabled  NCopyVariant=Disabled_SignalSpec  FilterICVariant=Disabled  IntegratorICVariant=InternalICs  ExternalResetVariant=Disabled  TRSumVariant=Passthrough  SumFdbkVariant=Disabled  SumVariant=Sum_PI  TsampFilterVariant=InternalTs  TsampNgainVariant=Passthrough  TsampIntegralVariant=Passthrough
  Saturation : Saturate  UpperLimit=4000  LowerLimit=-4000
  Scope : Scope
  Scope1 : Scope
  Sin : Subsystem
  Sin_(后续可换为轨迹规划结果前向角) : Subsystem
  Step : Subsystem
  beta : Scope  NumInputPorts=2
  rad1 : Constant  Value=v_obj
  方向盘转角 : Scope
  方向盘转角1 : Scope
  delta_sw : Outport
  T_vx : Outport  Port=2
  wires:
  Add/1 -> PID Controller/1
  vx_real/1 -> Gain/1, Scope1/1, Add/1
  PID Controller/1 -> Scope/1, Saturation/1
  Saturation/1 -> T_vx/1
  Step/1(delta_sw) -> 方向盘转角/1
  Sin_(后续可换为轨迹规划结果前向角)/1(delta_sw) -> 方向盘转角1/1, delta_sw/1
  Gain/1 -> beta/1
  Gain1/1 -> beta/2
  rad1/1 -> Gain1/1, Add/2

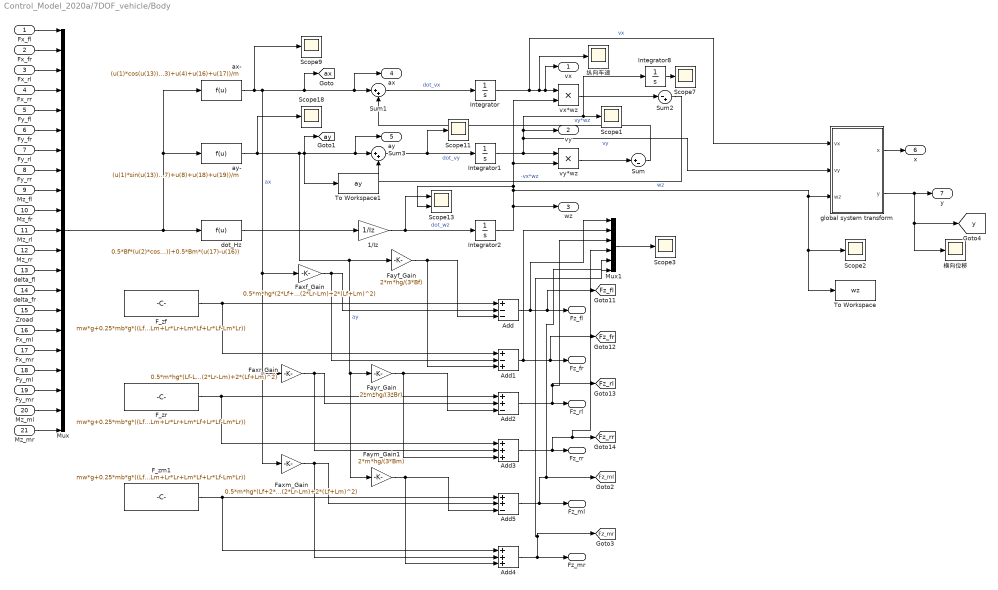
== system Control_Model_2020a/7DOF_vehicle/Body ==
  Fx_fl : Inport
  Fx_fr : Inport  Port=2
  Fx_rl : Inport  Port=3
  Fx_rr : Inport  Port=4
  Fy_fl : Inport  Port=5
  Fy_fr : Inport  Port=6
  Fy_rl : Inport  Port=7
  Fy_rr : Inport  Port=8
  Mz_fl : Inport  Port=9
  Mz_fr : Inport  Port=10
  Mz_rl : Inport  Port=11
  Mz_rr : Inport  Port=12
  delta_fl : Inport  Port=13
  delta_fr : Inport  Port=14
  Zroad : Inport  Port=15
  Fx_ml : Inport  Port=16
  Fx_mr : Inport  Port=17
  Fy_ml : Inport  Port=18
  Fy_mr : Inport  Port=19
  Mz_ml : Inport  Port=20
  Mz_mr : Inport  Port=21
  1/Iz : Gain  Gain=1/Iz
  Add : Sum  Inputs=+--
  Add1 : Sum  Inputs=+-+
  Add2 : Sum  Inputs=++-
  Add3 : Sum  Inputs=+++
  Add4 : Sum  Inputs=+++
  Add5 : Sum  Inputs=++-
  F_zf : Constant  Value=mw*g+0.25*mb*g*((Lf*Lr+Lm*Lf+Lm*Lm+Lr*Lr)/(Lf*Lf+Lm*Lm+Lr*Lr+Lm*Lf+Lr*Lf-Lm*Lr))
  F_zm1 : Constant  Value=mw*g+0.25*mb*g*((Lf*Lm-Lm*Lr+Lf*Lf+Lr*Lr)/(Lf*Lf+Lm*Lm+Lr*Lr+Lm*Lf+Lr*Lf-Lm*Lr))
  F_zr : Constant  Value=mw*g+0.25*mb*g*((Lf*Lr-Lm*Lr+Lm*Lm+Lf*Lf)/(Lf*Lf+Lm*Lm+Lr*Lr+Lm*Lf+Lr*Lf-Lm*Lr))
  Faxf_Gain : Gain  Gain=0.5*m*hg*(2*Lf+Lm+Lr)/((Lr-Lm)*(2*Lr-Lm)+2*(Lf+Lm)^2)
  Faxm_Gain : Gain  Gain=0.5*m*hg*(Lf+2*Lm-Lr)/((Lr-Lm)*(2*Lr-Lm)+2*(Lf+Lm)^2)
  Faxr_Gain : Gain  Gain=0.5*m*hg*(Lf-Lm+2*Lr)/((Lr-Lm)*(2*Lr-Lm)+2*(Lf+Lm)^2)
  Fayf_Gain : Gain  Gain=2*m*hg/(3*Bf)
  Faym_Gain1 : Gain  Gain=2*m*hg/(3*Bm)
  Fayr_Gain : Gain  Gain=2*m*hg/(3*Br)
  Integrator : Integrator  InitialCondition=vx0  LimitOutput=on  LowerSaturationLimit=0
  Integrator1 : Integrator
  Integrator2 : Integrator
  Integrator8 : Integrator
  Mux : Mux  Inputs=21
  Mux1 : Mux  Inputs=6
  Scope{1..3,7,9,11,18} (7 alike) : Scope
  Scope13 : Scope  NumInputPorts=2
  Sum : Sum  Inputs=|+-
  Sum1 : Sum  Inputs=|++
  Sum2 : Sum  Inputs=|-+
  Sum3 : Sum  Inputs=|++
  To Workspace : ToWorkspace  VariableName=wz  SaveFormat=Timeseries  SampleTime=-1
  To Workspace1 : ToWorkspace  VariableName=ay  SaveFormat=Timeseries  SampleTime=-1
  ax- : Fcn  Expr=(u(1)*cos(u(13))+u(2)*cos(u(14))-u(5)*sin(u(13))-u(6)*sin(u(14))+u(3)+u(4)+u(16)+u(17))/m
  ay- : Fcn  Expr=(u(1)*sin(u(13))+u(2)*sin(u(14))+u(5)*cos(u(13))+u(6)*cos(u(14))+u(7)+u(8)+u(18)+u(19))/m
  dot_Hz : Fcn  Expr=0.5*Bf*(u(2)*cos(u(14))-u(1)*cos(u(13))-u(6)*sin(u(14))+u(5)*sin(u(13)))+0.5*Br*(u(4)-u(3))+Lf*(u(1)*sin(u(13))+u(5)*cos(u(13))+u(2)*sin(u(14))+u(6)*cos(u(14)))-Lr*(u(7)+u(8))-Lm*(u(18)+u(19))+0.5*Bm*(u(17)-u(16))
  global system transform : Subsystem
  vx*wz : Product
  vy*wz : Product
  横向位移 : Scope
  纵向车速 : Scope
  vx : Outport
  vy : Outport  Port=2
  wz : Outport  Port=3
  ax : Outport  Port=4
  ay : Outport  Port=5
  x : Outport  Port=6
  y : Outport  Port=7
  Fz_fl : Outport  Port=8
  Fz_fr : Outport  Port=9
  Fz_rl : Outport  Port=10
  Fz_rr : Outport  Port=11
  Fz_ml : Outport  Port=12
  Fz_mr : Outport  Port=13
  tag scope: Fz_fl=global, Fz_fr=global, Fz_ml=global, Fz_mr=global, Fz_rl=global, Fz_rr=global, ax=global, ay=global, y=global
  wires:
  Integrator8/1 -> Scope7/1
  global system transform/2(y) -> y/1, [y], 横向位移/1
  global system transform/1(x) -> x/1
  Zroad/1 -> Mux/15
  Mux/1 -> dot_Hz/1, ay-/1, ax-/1
  delta_fr/1 -> Mux/14
  delta_fl/1 -> Mux/13
  Mz_rr/1 -> Mux/12
  Mz_fr/1 -> Mux/10
  Mz_fl/1 -> Mux/9
  Fy_rr/1 -> Mux/8
  Fy_rl/1 -> Mux/7
  Fy_fr/1 -> Mux/6
  Fy_fl/1 -> Mux/5
  Fx_rr/1 -> Mux/4
  Fx_rl/1 -> Mux/3
  Fx_fr/1 -> Mux/2
  Fx_fl/1 -> Mux/1
  Sum1/1 -> Integrator/1  "dot_vx"
  Integrator/1 -> 纵向车速/1, vx/1, vx*wz/1, global system transform/1(vx)  "vx"
  Integrator1/1 -> global system transform/2(vy), vy/1, Scope1/1, Integrator8/1, vy*wz/1  "vy"
  Sum3/1 -> Integrator1/1, Scope11/1  "dot_vy"
  1/Iz/1 -> Integrator2/1, Scope13/1  "dot_wz"
  Integrator2/1 -> Scope13/2, vy*wz/2, vx*wz/2, Scope2/1, To Workspace/1, global system transform/3(wz), wz/1  "wz"
  ay-/1 -> Scope18/1, ay/1, Sum3/1, To Workspace1/1, [ay], Faym_Gain1/1, Fayr_Gain/1, Fayf_Gain/1  "ay"
  vy*wz/1 -> Sum/1
  Sum/1 -> Sum1/2  "vy*wz"
  vx*wz/1 -> Sum2/1
  Sum2/1 -> Sum3/2  "-vx*wz"
  dot_Hz/1 -> 1/Iz/1
  ax-/1 -> Scope9/1, Faxm_Gain/1, Faxr_Gain/1, Faxf_Gain/1, ax/1, Sum1/1, [ax]  "ax"
  Add/1 -> Mux1/1, [Fz_fl], Fz_fl/1
  Add1/1 -> [Fz_fr], Fz_fr/1, Mux1/2
  Add2/1 -> Mux1/3, [Fz_rl], Fz_rl/1
  Add3/1 -> Fz_rr/1, Mux1/4, [Fz_rr]
  Mux1/1 -> Scope3/1
  Mz_rl/1 -> Mux/11
  Fx_ml/1 -> Mux/16
  Fx_mr/1 -> Mux/17
  Fy_ml/1 -> Mux/18
  Fy_mr/1 -> Mux/19
  Mz_ml/1 -> Mux/20
  Mz_mr/1 -> Mux/21
  F_zf/1 -> Add1/1, Add/1
  Faxf_Gain/1 -> Add1/2, Add/2
  Fayf_Gain/1 -> Add1/3, Add/3
  Faxr_Gain/1 -> Add3/2, Add2/2
  Fayr_Gain/1 -> Add3/3, Add2/3
  F_zr/1 -> Add3/1, Add2/1
  F_zm1/1 -> Add4/1, Add5/1
  Faxm_Gain/1 -> Add4/2, Add5/2
  Faym_Gain1/1 -> Add4/3, Add5/3
  Add5/1 -> Mux1/5, [Fz_ml], Fz_ml/1
  Add4/1 -> Mux1/6, [Fz_mr], Fz_mr/1

== system Control_Model_2020a/7DOF_vehicle/Steering ==
  delta_sw : Inport
  Add : Sum
  Add2 : Sum  Inputs=-+
  Add3 : Sum
  Constant : Constant  Value=Lr
  Constant1 : Constant  Value=Lf
  Constant2 : Constant  Value=i_sw
  Constant3 : Constant  Value=Br
  Divide : Product  Inputs=*/
  Divide1 : Product  Inputs=/*
  Divide2 : Product  Inputs=/*
  Gain : Gain  Gain=2
  Product : Product
  Product1 : Product
  Trigonometric Function : Trigonometry  Operator=atan
  Trigonometric Function1 : Trigonometry  Operator=tan
  Trigonometric Function2 : Trigonometry  Operator=atan
  test1 : Scope
  test2 : Scope  NumInputPorts=2
  delta_fl : Outport
  delta_fr : Outport  Port=2
  delta_s : Outport  Port=3
  wires:
  Trigonometric Function2/1 -> test2/1, delta_fr/1
  Divide2/1 -> Trigonometric Function2/1
  Add3/1 -> Divide2/1
  Trigonometric Function/1 -> test2/2, delta_fl/1
  Divide1/1 -> Trigonometric Function/1
  Product/1 -> Divide1/2, Divide2/2
  Add2/1 -> Divide1/1
  Product1/1 -> Add2/1, Add3/1
  Constant3/1 -> Product1/1
  Gain/1 -> Add2/2, Add3/2, Product/2
  Trigonometric Function1/1 -> Product1/2, Product/1
  Divide/1 -> test1/1, delta_s/1, Trigonometric Function1/1  "delta_s"
  Constant2/1 -> Divide/2
  delta_sw/1 -> Divide/1
  Add/1 -> Gain/1
  Constant/1 -> Add/2
  Constant1/1 -> Add/1

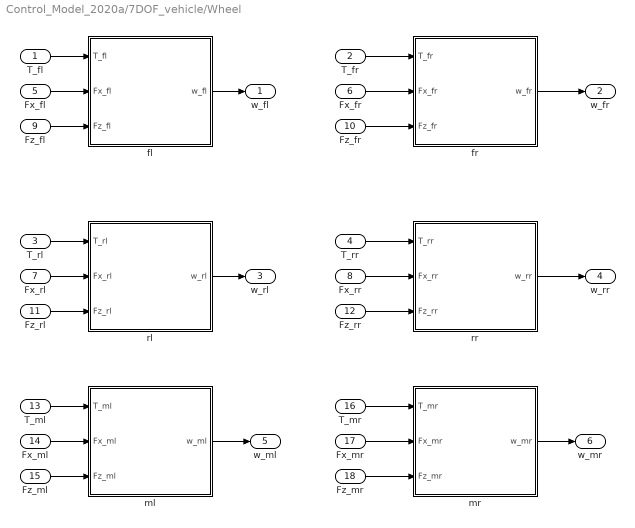
== system Control_Model_2020a/7DOF_vehicle/Wheel ==
  T_fl : Inport
  T_fr : Inport  Port=2
  T_rl : Inport  Port=3
  T_rr : Inport  Port=4
  Fx_fl : Inport  Port=5
  Fx_fr : Inport  Port=6
  Fx_rl : Inport  Port=7
  Fx_rr : Inport  Port=8
  Fz_fl : Inport  Port=9
  Fz_fr : Inport  Port=10
  Fz_rl : Inport  Port=11
  Fz_rr : Inport  Port=12
  T_ml : Inport  Port=13
  Fx_ml : Inport  Port=14
  Fz_ml : Inport  Port=15
  T_mr : Inport  Port=16
  Fx_mr : Inport  Port=17
  Fz_mr : Inport  Port=18
  fl : Subsystem
  fr : Subsystem
  ml : Subsystem
  mr : Subsystem
  rl : Subsystem
  rr : Subsystem
  w_fl : Outport
  w_fr : Outport  Port=2
  w_rl : Outport  Port=3
  w_rr : Outport  Port=4
  w_ml : Outport  Port=5
  w_mr : Outport  Port=6
  wires:
  T_fl/1 -> fl/1(T_fl)
  Fx_fl/1 -> fl/2(Fx_fl)
  Fz_fl/1 -> fl/3(Fz_fl)
  fl/1(w_fl) -> w_fl/1
  fr/1(w_fr) -> w_fr/1
  T_fr/1 -> fr/1(T_fr)
  Fx_fr/1 -> fr/2(Fx_fr)
  Fz_fr/1 -> fr/3(Fz_fr)
  T_rl/1 -> rl/1(T_rl)
  Fx_rl/1 -> rl/2(Fx_rl)
  Fz_rl/1 -> rl/3(Fz_rl)
  rl/1(w_rl) -> w_rl/1
  T_rr/1 -> rr/1(T_rr)
  Fx_rr/1 -> rr/2(Fx_rr)
  Fz_rr/1 -> rr/3(Fz_rr)
  rr/1(w_rr) -> w_rr/1
  T_mr/1 -> mr/1(T_mr)
  Fx_mr/1 -> mr/2(Fx_mr)
  Fz_mr/1 -> mr/3(Fz_mr)
  T_ml/1 -> ml/1(T_ml)
  Fx_ml/1 -> ml/2(Fx_ml)
  Fz_ml/1 -> ml/3(Fz_ml)
  ml/1(w_ml) -> w_ml/1
  mr/1(w_mr) -> w_mr/1

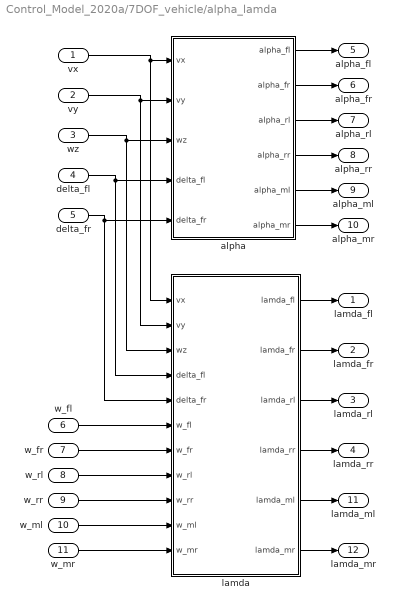
== system Control_Model_2020a/7DOF_vehicle/alpha_lamda ==
  vx : Inport
  vy : Inport  Port=2
  wz : Inport  Port=3
  delta_fl : Inport  Port=4
  delta_fr : Inport  Port=5
  w_fl : Inport  Port=6
  w_fr : Inport  Port=7
  w_rl : Inport  Port=8
  w_rr : Inport  Port=9
  w_ml : Inport  Port=10
  w_mr : Inport  Port=11
  alpha : Subsystem
  lamda : Subsystem
  lamda_fl : Outport
  lamda_fr : Outport  Port=2
  lamda_rl : Outport  Port=3
  lamda_rr : Outport  Port=4
  alpha_fl : Outport  Port=5
  alpha_fr : Outport  Port=6
  alpha_rl : Outport  Port=7
  alpha_rr : Outport  Port=8
  alpha_ml : Outport  Port=9
  alpha_mr : Outport  Port=10
  lamda_ml : Outport  Port=11
  lamda_mr : Outport  Port=12
  wires:
  lamda/3(lamda_rl) -> lamda_rl/1
  lamda/4(lamda_rr) -> lamda_rr/1
  lamda/2(lamda_fr) -> lamda_fr/1
  lamda/1(lamda_fl) -> lamda_fl/1
  w_rr/1 -> lamda/9(w_rr)
  w_rl/1 -> lamda/8(w_rl)
  w_fr/1 -> lamda/7(w_fr)
  w_fl/1 -> lamda/6(w_fl)
  delta_fr/1 -> alpha/5(delta_fr), lamda/5(delta_fr)
  delta_fl/1 -> alpha/4(delta_fl), lamda/4(delta_fl)
  wz/1 -> alpha/3(wz), lamda/3(wz)
  vy/1 -> alpha/2(vy), lamda/2(vy)
  vx/1 -> alpha/1(vx), lamda/1(vx)
  alpha/4(alpha_rr) -> alpha_rr/1
  alpha/3(alpha_rl) -> alpha_rl/1
  alpha/2(alpha_fr) -> alpha_fr/1
  alpha/1(alpha_fl) -> alpha_fl/1
  alpha/5(alpha_ml) -> alpha_ml/1
  alpha/6(alpha_mr) -> alpha_mr/1
  lamda/5(lamda_ml) -> lamda_ml/1
  lamda/6(lamda_mr) -> lamda_mr/1
  w_ml/1 -> lamda/10(w_ml)
  w_mr/1 -> lamda/11(w_mr)

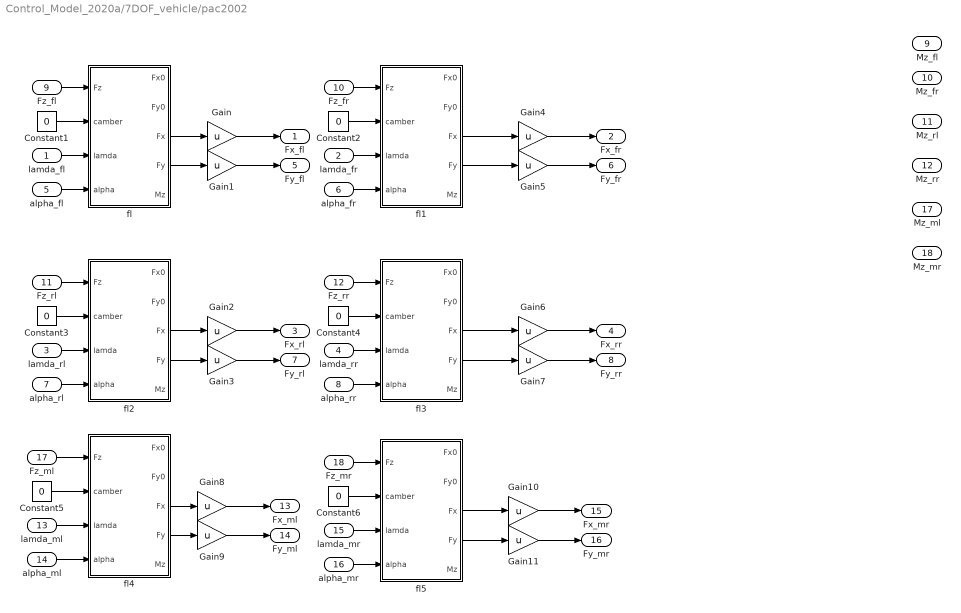
== system Control_Model_2020a/7DOF_vehicle/pac2002 ==
  lamda_fl : Inport
  lamda_fr : Inport  Port=2
  lamda_rl : Inport  Port=3
  lamda_rr : Inport  Port=4
  alpha_fl : Inport  Port=5
  alpha_fr : Inport  Port=6
  alpha_rl : Inport  Port=7
  alpha_rr : Inport  Port=8
  Fz_fl : Inport  Port=9
  Fz_fr : Inport  Port=10
  Fz_rl : Inport  Port=11
  Fz_rr : Inport  Port=12
  lamda_ml : Inport  Port=13
  alpha_ml : Inport  Port=14
  lamda_mr : Inport  Port=15
  alpha_mr : Inport  Port=16
  Fz_ml : Inport  Port=17
  Fz_mr : Inport  Port=18
  Constant{1..6} (6 alike) : Constant  Value=0
  Gain{,1..11} (12 alike) : Gain  Gain=u
  fl : MATLAB Function  TreatAsAtomicUnit=on
  fl1 : MATLAB Function  TreatAsAtomicUnit=on
  fl2 : MATLAB Function  TreatAsAtomicUnit=on
  fl3 : MATLAB Function  TreatAsAtomicUnit=on
  fl4 : MATLAB Function  TreatAsAtomicUnit=on
  fl5 : MATLAB Function  TreatAsAtomicUnit=on
  Fx_fl : Outport
  Fx_fr : Outport  Port=2
  Fx_rl : Outport  Port=3
  Fx_rr : Outport  Port=4
  Fy_fl : Outport  Port=5
  Fy_fr : Outport  Port=6
  Fy_rl : Outport  Port=7
  Fy_rr : Outport  Port=8
  Mz_fl : Outport  Port=9
  Mz_fr : Outport  Port=10
  Mz_rl : Outport  Port=11
  Mz_rr : Outport  Port=12
  Fx_ml : Outport  Port=13
  Fy_ml : Outport  Port=14
  Fx_mr : Outport  Port=15
  Fy_mr : Outport  Port=16
  Mz_ml : Outport  Port=17
  Mz_mr : Outport  Port=18
  wires:
  fl1/3(Fx) -> Gain4/1
  fl2/4(Fy) -> Gain3/1
  fl2/3(Fx) -> Gain2/1
  fl3/4(Fy) -> Gain7/1
  fl3/3(Fx) -> Gain6/1
  fl1/4(Fy) -> Gain5/1
  fl/4(Fy) -> Gain1/1
  fl/3(Fx) -> Gain/1
  lamda_fl/1 -> fl/3(lamda)
  alpha_fl/1 -> fl/4(alpha)
  Fz_fl/1 -> fl/1(Fz)
  Constant1/1 -> fl/2(camber)
  lamda_fr/1 -> fl1/3(lamda)
  alpha_fr/1 -> fl1/4(alpha)
  Fz_fr/1 -> fl1/1(Fz)
  lamda_rl/1 -> fl2/3(lamda)
  alpha_rl/1 -> fl2/4(alpha)
  Fz_rl/1 -> fl2/1(Fz)
  lamda_rr/1 -> fl3/3(lamda)
  alpha_rr/1 -> fl3/4(alpha)
  Fz_rr/1 -> fl3/1(Fz)
  Constant2/1 -> fl1/2(camber)
  Constant3/1 -> fl2/2(camber)
  Constant4/1 -> fl3/2(camber)
  Gain1/1 -> Fy_fl/1
  Gain2/1 -> Fx_rl/1
  Gain3/1 -> Fy_rl/1
  Gain4/1 -> Fx_fr/1
  Gain5/1 -> Fy_fr/1
  Gain6/1 -> Fx_rr/1
  Gain7/1 -> Fy_rr/1
  Gain/1 -> Fx_fl/1
  Fz_ml/1 -> fl4/1(Fz)
  Constant5/1 -> fl4/2(camber)
  lamda_ml/1 -> fl4/3(lamda)
  alpha_ml/1 -> fl4/4(alpha)
  Fz_mr/1 -> fl5/1(Fz)
  Constant6/1 -> fl5/2(camber)
  lamda_mr/1 -> fl5/3(lamda)
  alpha_mr/1 -> fl5/4(alpha)
  Gain8/1 -> Fx_ml/1
  Gain9/1 -> Fy_ml/1
  fl4/3(Fx) -> Gain8/1
  fl4/4(Fy) -> Gain9/1
  Gain10/1 -> Fx_mr/1
  Gain11/1 -> Fy_mr/1
  fl5/3(Fx) -> Gain10/1
  fl5/4(Fy) -> Gain11/1

== system Control_Model_2020a/7DOF_vehicle/rad//s_to_rpm ==
  w_fl : Inport
  w_fr : Inport  Port=2
  w_rl : Inport  Port=3
  w_rr : Inport  Port=4
  w_ml : Inport  Port=5
  w_mr : Inport  Port=6
  Gain{,1..5} (6 alike) : Gain  Gain=30/pi
  n_fl : Outport
  n_fr : Outport  Port=2
  n_rl : Outport  Port=3
  n_rr : Outport  Port=4
  n_ml : Outport  Port=5
  n_mr : Outport  Port=6
  wires:
  Gain3/1 -> n_rr/1
  Gain1/1 -> n_fr/1
  Gain2/1 -> n_rl/1
  w_rr/1 -> Gain3/1
  w_rl/1 -> Gain2/1
  w_fr/1 -> Gain1/1
  Gain/1 -> n_fl/1
  w_fl/1 -> Gain/1
  w_ml/1 -> Gain4/1
  w_mr/1 -> Gain5/1
  Gain4/1 -> n_ml/1
  Gain5/1 -> n_mr/1

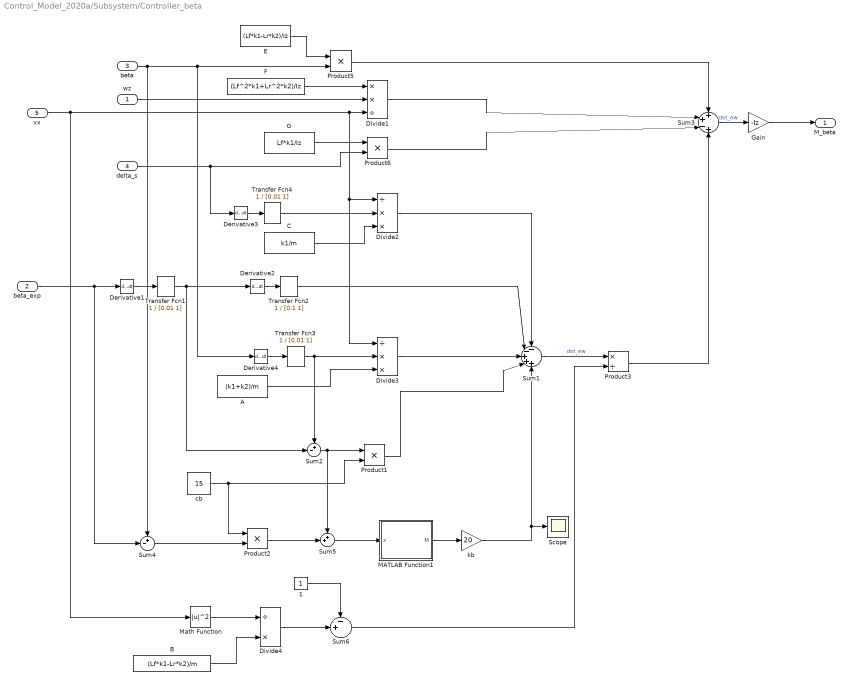
== system Control_Model_2020a/Subsystem/Controller_beta ==
  wz : Inport
  beta_exp : Inport  Port=2
  beta : Inport  Port=3
  delta_s : Inport  Port=4
  vx : Inport  Port=5
  1 : Constant
  A : Constant  Value=(k1+k2)/m
  B : Constant  Value=(Lf*k1-Lr*k2)/m
  C : Constant  Value=k1/m
  Derivative{1..4} (4 alike) : Derivative
  Divide1 : Product  Inputs=**/
  Divide2 : Product  Inputs=/**
  Divide3 : Product  Inputs=/**
  Divide4 : Product  Inputs=/*
  E : Constant  Value=(Lf*k1-Lr*k2)/Iz
  F : Constant  Value=(Lf^2*k1+Lr^2*k2)/Iz
  G : Constant  Value=Lf*k1/Iz
  Gain : Gain  Gain=-Iz
  MATLAB Function1 : MATLAB Function  TreatAsAtomicUnit=on
  Math Function : Math  Operator=magnitude^2  SignedPower=on  SaturateOnIntegerOverflow=on
  Product{1..2,5..6} (4 alike) : Product
  Product3 : Product  Inputs=*/
  Scope : Scope
  Sum1 : Sum  Inputs=--+++
  Sum2 : Sum  Inputs=+-|
  Sum3 : Sum  Inputs=++-+
  Sum4 : Sum  Inputs=+-|
  Sum5 : Sum  Inputs=++|
  Sum6 : Sum  Inputs=-+|
  Transfer Fcn1 : TransferFcn  Numerator=1  Denominator=[0.01 1]
  Transfer Fcn2 : TransferFcn  Numerator=1  Denominator=[0.1 1]
  Transfer Fcn3 : TransferFcn  Numerator=1  Denominator=[0.01 1]
  Transfer Fcn4 : TransferFcn  Numerator=1  Denominator=[0.01 1]
  cb : Constant  Value=15
  kb : Gain  Gain=20
  M_beta : Outport
  wires:
  Gain/1 -> M_beta/1
  wz/1 -> Divide1/2
  beta/1 -> Derivative4/1, Product5/2, Sum4/1
  E/1 -> Product5/1
  F/1 -> Divide1/1
  vx/1 -> Math Function/1, Divide3/1, Divide2/1, Divide1/3
  G/1 -> Product6/1
  delta_s/1 -> Derivative3/1, Product6/2
  Product5/1 -> Sum3/1
  Divide1/1 -> Sum3/2
  Product6/1 -> Sum3/3
  Derivative3/1 -> Transfer Fcn4/1
  C/1 -> Divide2/3
  Transfer Fcn4/1 -> Divide2/2
  Divide2/1 -> Sum1/1
  Sum3/1 -> Gain/1  "dot_ew"
  beta_exp/1 -> Derivative1/1, Sum4/2
  Derivative1/1 -> Transfer Fcn1/1
  Derivative2/1 -> Transfer Fcn2/1
  Transfer Fcn2/1 -> Sum1/2
  A/1 -> Divide3/3
  Derivative4/1 -> Transfer Fcn3/1
  Transfer Fcn3/1 -> Divide3/2, Sum2/1
  Divide3/1 -> Sum1/3
  Sum2/1 -> Product1/1, Sum5/1
  cb/1 -> Product1/2, Product2/1
  Product1/1 -> Sum1/4
  Sum4/1 -> Product2/2
  Product2/1 -> Sum5/2
  Sum5/1 -> MATLAB Function1/1(x)
  MATLAB Function1/1(M) -> kb/1
  kb/1 -> Scope/1, Sum1/5
  B/1 -> Divide4/2
  Math Function/1 -> Divide4/1
  Divide4/1 -> Sum6/2
  1/1 -> Sum6/1
  Sum1/1 -> Product3/1  "dot_ew"
  Sum6/1 -> Product3/2
  Product3/1 -> Sum3/4
  Transfer Fcn1/1 -> Derivative2/1, Sum2/2

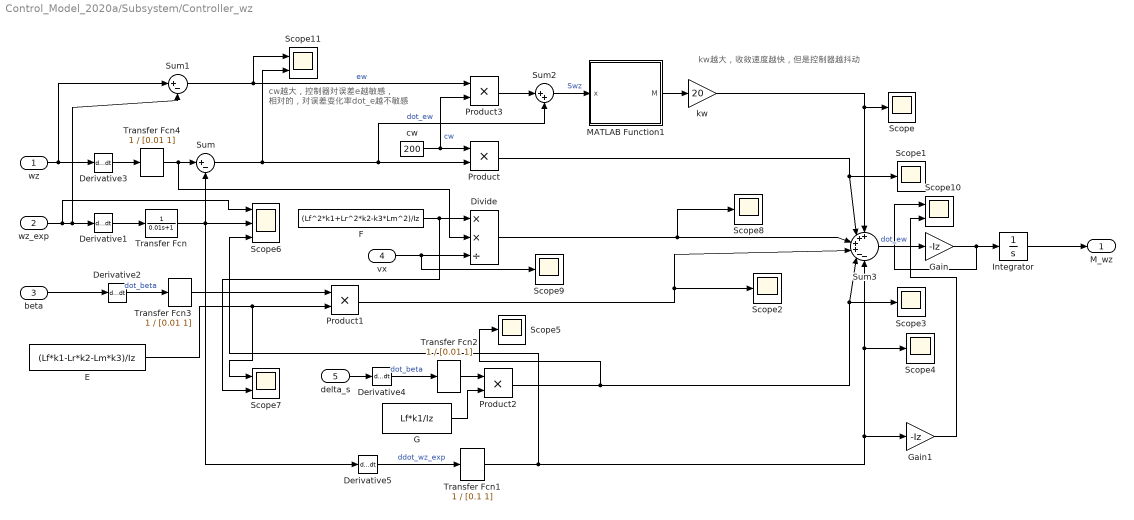
== system Control_Model_2020a/Subsystem/Controller_wz ==
  note: kw越大，收敛速度越快，但是控制器越抖动
  note: cw越大，控制器对误差e越敏感，
      | 相对的，对误差变化率dot_e越不敏感
  wz : Inport
  wz_exp : Inport  Port=2
  beta : Inport  Port=3
  vx : Inport  Port=4
  delta_s : Inport  Port=5
  Derivative{1..5} (5 alike) : Derivative
  Divide : Product  Inputs=**/
  E : Constant  Value=(Lf*k1-Lr*k2-Lm*k3)/Iz
  F : Constant  Value=(Lf^2*k1+Lr^2*k2-k3*Lm^2)/Iz
  G : Constant  Value=Lf*k1/Iz
  Gain : Gain  Gain=-Iz
  Gain1 : Gain  Gain=-Iz
  Integrator : Integrator
  MATLAB Function1 : MATLAB Function  TreatAsAtomicUnit=on
  Product{,1..3} (4 alike) : Product
  Scope{,1..5,8..9} (8 alike) : Scope
  Scope10 : Scope  NumInputPorts=2
  Scope11 : Scope  NumInputPorts=2
  Scope6 : Scope  NumInputPorts=3
  Scope7 : Scope  NumInputPorts=2
  Sum : Sum  Inputs=|+-
  Sum1 : Sum  Inputs=|+-
  Sum2 : Sum  Inputs=|++
  Sum3 : Sum  Inputs=++++--
  Transfer Fcn{,2..4} (4 alike) : TransferFcn  Numerator=1  Denominator=[0.01 1]
  Transfer Fcn1 : TransferFcn  Numerator=1  Denominator=[0.1 1]
  cw : Constant  Value=200
  kw : Gain  Gain=20
  M_wz : Outport
  wires:
  cw/1 -> Product3/2, Product/1  "cw"
  wz_exp/1 -> Scope6/1, Derivative1/1, Sum1/2
  Derivative1/1 -> Transfer Fcn/1
  beta/1 -> Derivative2/1
  wz/1 -> Derivative3/1, Sum1/1
  Transfer Fcn4/1 -> Divide/2, Sum/1
  Sum/1 -> Sum2/2, Product/2, Scope11/2  "dot_ew"
  Derivative2/1 -> Transfer Fcn3/1  "dot_beta"
  E/1 -> Scope7/1, Product1/2
  F/1 -> Scope7/2, Divide/1
  vx/1 -> Scope9/1, Divide/3
  delta_s/1 -> Derivative4/1
  Derivative4/1 -> Transfer Fcn2/1  "dot_beta"
  G/1 -> Product2/2
  Sum1/1 -> Scope11/1, Product3/1  "ew"
  Product3/1 -> Sum2/1
  Sum2/1 -> MATLAB Function1/1(x)  "Swz"
  MATLAB Function1/1(M) -> kw/1
  Derivative5/1 -> Transfer Fcn1/1  "ddot_wz_exp"
  kw/1 -> Sum3/1, Scope/1
  Product/1 -> Sum3/2, Scope1/1
  Divide/1 -> Scope8/1, Sum3/3
  Product1/1 -> Sum3/4, Scope2/1
  Product2/1 -> Scope5/1, Scope3/1, Sum3/5
  Sum3/1 -> Gain/1  "dot_ew"
  Gain/1 -> Scope10/1, Integrator/1
  Transfer Fcn/1 -> Derivative5/1, Scope6/2, Sum/2
  Transfer Fcn1/1 -> Scope6/3, Gain1/1, Sum3/6, Scope4/1
  Transfer Fcn2/1 -> Product2/1
  Transfer Fcn3/1 -> Product1/1
  Derivative3/1 -> Transfer Fcn4/1
  Integrator/1 -> M_wz/1
  Gain1/1 -> Scope10/2

== system Control_Model_2020a/Subsystem/Union_Control ==
  beta : Inport
  u : Inport  Port=2
  Abs : Abs
  Derivative2 : Derivative
  Divide : Product  Inputs=*/
  Gain : Gain  Gain=57
  Gain1 : Gain  Gain=57
  MATLAB Function1 : MATLAB Function  TreatAsAtomicUnit=on
  Product : Product
  Saturation : Saturate  UpperLimit=1  LowerLimit=0
  Scope : Scope
  Scope1 : Scope
  Scope2 : Scope
  Sum2 : Sum  Inputs=++|
  Transfer Fcn3 : TransferFcn  Numerator=1  Denominator=[0.01 1]
  p : Outport
  wires:
  Product/1 -> Sum2/2
  Transfer Fcn3/1 -> Gain1/1
  beta/1 -> Derivative2/1, Gain/1
  Derivative2/1 -> Transfer Fcn3/1  "dot_beta"
  Saturation/1 -> Scope2/1, p/1
  MATLAB Function1/1(B1) -> Product/2
  Sum2/1 -> Abs/1  "Swz"
  u/1 -> MATLAB Function1/1(u)
  Divide/1 -> Saturation/1, Scope1/1
  MATLAB Function1/2(B2) -> Divide/2
  Abs/1 -> Scope/1, Divide/1
  Gain/1 -> Sum2/1
  Gain1/1 -> Product/1

== system Control_Model_2020a/开环驾驶员模型/DLC ==
  Clock{,1..3} (4 alike) : Clock
  Constant : Constant  Value=0
  Constant1 : Constant  Value=0
  Gain : Gain  Gain=-1
  Scope : Scope
  Switch : Switch  Criteria=u2 > Threshold  Threshold=3
  Switch1 : Switch  Criteria=u2 > Threshold  Threshold=7
  Switch2 : Switch  Criteria=u2 > Threshold  Threshold=8
  Switch3 : Switch  Criteria=u2 > Threshold  Threshold=12
  Transport Delay1 : TransportDelay  DelayTime=3
  rad : Sin  Amplitude=2  Frequency=pi/2  SampleTime=0
  rad1 : Sin  Amplitude=2  Frequency=pi/2  SampleTime=0
  delta_sw : Outport
  wires:
  Constant/1 -> Switch/3
  Transport Delay1/1 -> Scope/1, Switch/1
  Switch/1 -> Switch1/3
  Clock1/1 -> Switch1/2
  rad/1 -> Transport Delay1/1
  Clock/1 -> Switch/2
  Constant1/1 -> Switch1/1
  Clock2/1 -> Switch2/2
  Switch1/1 -> Switch2/3
  rad1/1 -> Gain/1
  Gain/1 -> Switch2/1
  Switch2/1 -> Switch3/3
  Clock3/1 -> Switch3/2
  Switch3/1 -> delta_sw/1

== system Control_Model_2020a/开环驾驶员模型/Sin ==
  Degrees to Radians : simulink_extras/Transformations/Degrees to Radians
  Gain : Gain
  Scope1 : Scope
  Signal Builder : Subsystem  Tag=STV Subsys  LoadFcn=sigbuilder_block('load');  StartFcn=sigbuilder_block('start');  StopFcn=sigbuilder_block('stop');  ClipboardFcn=sigbuilder_block('clipboard');  mask(Sigbuilder block){tuvar=[0:10]}
      mask help: Simulink:masks:SigbuilderBlock_MD
      mask init:
      | if ~strcmp(get_param(bdroot(gcbh),'SimulationStatus'),'stopped') tuvar = sigbuilder_block('maskInit'); end
      settings: CopyFcn=sigbuilder_block('copy');  DeleteFcn=sigbuilder_block('delete');  ModelCloseFcn=sigbuilder_block('modelClose');  PreSaveFcn=sigbuilder_block('preSave');  PauseFcn=sigbuilder_block('pause');  ContinueFcn=sigbuilder_block('continue');  NameChangeFcn=sigbuilder_block('namechange');  OpenFcn=sigbuilder_block('open',[837.75 230.25 550.5 399.75 ]);  CloseFcn=sigbuilder_block('close');
      mask Display: plot(0, 0, 100, 100,[2, 2, 32, 32, 2], [68, 8, 8, 68, 68],[32, 2], [38, 38], [32, 19, 2],[53, 60, 44], [32, 17, 17, 2],[16, 16, 31, 31]);txt = getActiveGroup(gcbh);text(2, 100, txt,'verticalAlignment', 'top');
  Out1 : Outport
  wires:
  Signal Builder/1(Signal 1) -> Degrees to Radians/1
  Degrees to Radians/1 -> Gain/1
  Gain/1 -> Scope1/1, Out1/1
